simulink model "driveControl_StateflowChart139"  (R2023a)
settings: Solver=VariableStepAuto  StartTime=0.0  StopTime=10.0  RelTol=1e-3
settings Model: Creator=Franz  LastModifiedBy=Franz

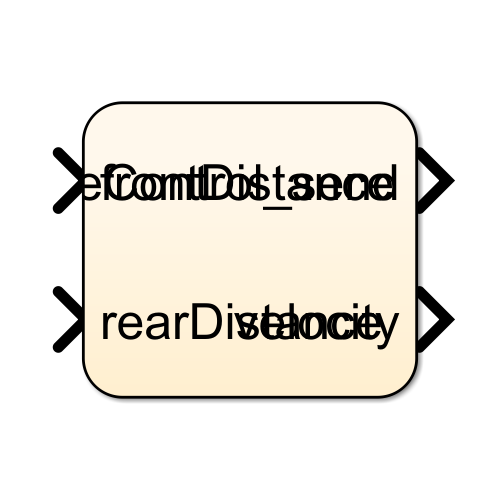
[thumbnail: Simulink's stored preview of the top-level diagram]
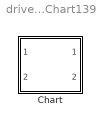
== system driveControl_StateflowChart139 ==
  Chart : Stateflow chart  TreatAsAtomicUnit=on

== stateflow chart driveControl_StateflowChart139/Chart ==
  state chart
    state chartRegion [parallel]
      settings: executionOrder=1
      state DriveControlComponent
        state driveControlPort [parallel]
          settings: executionOrder=1
          state Idle
          state WaitforCoordinator
          state WaitForOvertaking
          (default) -> Idle
          WaitForOvertaking -> Idle : [communicator_recv == 2]{send(executedOvertaking.overtakingInitPort);}
          WaitforCoordinator -> WaitForOvertaking [order 2] : grantPermission{communicator_send = 1;}
          WaitforCoordinator -> Idle [order 1] : denyPermission{communicator_send = 4;}
          Idle -> WaitforCoordinator : [communicator_recv==1]{send(OvertakingRequested,overtkingIniPort), coordination_Successfull = true;}
        state driving [parallel]
          settings: executionOrder=2
      (default) -> DriveControlComponent
  (default) -> chart
  data: frontDistance input Int32; rearDistance input; driveControl_send output; velocity output
